simulink model "bike_model_v1_20190531_oldmodel_positionfeedback"  (R2016b)
settings: Solver=ode23s  StartTime=0.0  StopTime=sim_time  FixedStep=Ts_IMU  MaxStep=Ts  RelTol=1e-3
values from neighbouring files (symbols this model uses):
  A = [0      0            1 ... (first row only)    [bike_init_v1_20190528_oldmodel_positionfeedback_and_indicator.m]    (also in bike_init_v1_20190531_oldmodel_positionfeedback_and_indicator.m)
  A_kalman = [1 0 Ts 0; 0 1 0 Ts; 0 0 1 0; 0 0 0 1]    [bike_init_v1_20190528_oldmodel_positionfeedback_and_indicator.m]    (also in bike_init_v1_20190531_oldmodel_positionfeedback_and_indicator.m)
  a_real = b_real-0.77    (= 0.325)    [bike_init_v1_20190528_oldmodel_positionfeedback_and_indicator.m]    (also in bike_init_v1_20190531_oldmodel_positionfeedback_and_indicator.m)
  B = [0; 1; (a_real*v*sin(lambda_real))/(h_real*b_real)]    [bike_init_v1_20190528_oldmodel_positionfeedback_and_indicator.m]    (also in bike_init_v1_20190531_oldmodel_positionfeedback_and_indicator.m)
  B_kalman = [0 0 0 0; 0 0 0 0; 0 0 0 0; 0 0 0 0]    [bike_init_v1_20190528_oldmodel_positionfeedback_and_indicator.m]    (also in bike_init_v1_20190531_oldmodel_positionfeedback_and_indicator.m)
  b_model = 1.095    [bike_init_v1_20190528_oldmodel_positionfeedback_and_indicator.m]    (also in bike_init_v1_20190531_oldmodel_positionfeedback_and_indicator.m)
  b_real = 1.095    [bike_init_v1_20190528_oldmodel_positionfeedback_and_indicator.m]    (also in bike_init_v1_20190531_oldmodel_positionfeedback_and_indicator.m)
  C = eye(3)    [bike_init_v1_20190528_oldmodel_positionfeedback_and_indicator.m]    (also in bike_init_v1_20190531_oldmodel_positionfeedback_and_indicator.m)
  C_kalman = [1 0 0 0; 0 1 0 0; 0 0 1 0; 0 0 0 1]    [bike_init_v1_20190528_oldmodel_positionfeedback_and_indicator.m]    (also in bike_init_v1_20190531_oldmodel_positionfeedback_and_indicator.m)
  complementary = 0.985    [bike_init_v1_20190528_oldmodel_positionfeedback_and_indicator.m]    (also in bike_init_v1_20190531_oldmodel_positionfeedback_and_indicator.m)
  cumulative_dist_along_path = [0;cumsum(dist_from_vertex_to_vertex,1)]    [bike_init_v1_20190528_oldmodel_positionfeedback_and_indicator.m]    (also in bike_init_v1_20190531_oldmodel_positionfeedback_and_indicator.m)
  D = zeros(3,1)    [bike_init_v1_20190528_oldmodel_positionfeedback_and_indicator.m]    (also in bike_init_v1_20190531_oldmodel_positionfeedback_and_indicator.m)
  D_kalman = [0 0 0 0; 0 0 0 0; 0 0 0 0; 0 0 0 0]    [bike_init_v1_20190528_oldmodel_positionfeedback_and_indicator.m]    (also in bike_init_v1_20190531_oldmodel_positionfeedback_and_indicator.m)
  damp = 0.4    [bike_init_v1_20190528_oldmodel_positionfeedback_and_indicator.m]    (also in bike_init_v1_20190531_oldmodel_positionfeedback_and_indicator.m)
  Dead_Band = [0.055,-0.055,0.005]    [bike_init_v1_20190528_oldmodel_positionfeedback_and_indicator.m]    (also in bike_init_v1_20190531_oldmodel_positionfeedback_and_indicator.m)
  delay = 0.045    [bike_init_v1_20190528_oldmodel_positionfeedback_and_indicator.m]    (also in bike_init_v1_20190531_oldmodel_positionfeedback_and_indicator.m)
  delta_control = 1    [bike_init_v1_20190528_oldmodel_positionfeedback_and_indicator.m]    (also in bike_init_v1_20190531_oldmodel_positionfeedback_and_indicator.m)
  direct_control = 1    [bike_init_v1_20190528_oldmodel_positionfeedback_and_indicator.m]    (also in bike_init_v1_20190531_oldmodel_positionfeedback_and_indicator.m)
  filter_model = 1    [bike_init_v1_20190528_oldmodel_positionfeedback_and_indicator.m]    (also in bike_init_v1_20190531_oldmodel_positionfeedback_and_indicator.m)
  forward_motor_dynamics = 0    [bike_init_v1_20190528_oldmodel_positionfeedback_and_indicator.m]    (also in bike_init_v1_20190531_oldmodel_positionfeedback_and_indicator.m)
  fr_oscil = 1    [bike_init_v1_20190528_oldmodel_positionfeedback_and_indicator.m]    (also in bike_init_v1_20190531_oldmodel_positionfeedback_and_indicator.m)
  g = 9.81    [bike_init_v1_20190528_oldmodel_positionfeedback_and_indicator.m]    (also in bike_init_v1_20190531_oldmodel_positionfeedback_and_indicator.m)
  gain = 0.3    [bike_init_v1_20190528_oldmodel_positionfeedback_and_indicator.m]    (also in bike_init_v1_20190531_oldmodel_positionfeedback_and_indicator.m)
  h_real = 0.586    [bike_init_v1_20190528_oldmodel_positionfeedback_and_indicator.m]    (also in bike_init_v1_20190531_oldmodel_positionfeedback_and_indicator.m)
  IMU_height_model = 0.45    [bike_init_v1_20190528_oldmodel_positionfeedback_and_indicator.m]    (also in bike_init_v1_20190531_oldmodel_positionfeedback_and_indicator.m)
  IMU_height_real = 0.45    [bike_init_v1_20190528_oldmodel_positionfeedback_and_indicator.m]    (also in bike_init_v1_20190531_oldmodel_positionfeedback_and_indicator.m)
  initial_states = [deg2rad(0) deg2rad(0) deg2rad(0)]    [bike_init_v1_20190528_oldmodel_positionfeedback_and_indicator.m]    (also in bike_init_v1_20190531_oldmodel_positionfeedback_and_indicator.m = [deg2rad(2) deg2rad(0) deg2rad(0)])
  initial_x = path_x(1)+x_ini_diff    [bike_init_v1_20190528_oldmodel_positionfeedback_and_indicator.m]    (also in bike_init_v1_20190531_oldmodel_positionfeedback_and_indicator.m = 0)
  initial_y = radius+y_ini_diff    (= 20)    [bike_init_v1_20190528_oldmodel_positionfeedback_and_indicator.m]    (also in bike_init_v1_20190531_oldmodel_positionfeedback_and_indicator.m = 0)
  input_velocity = 7    [bike_init_v1_20190528_oldmodel_positionfeedback_and_indicator.m]    (also in bike_init_v1_20190531_oldmodel_positionfeedback_and_indicator.m = 3)
  K_full_dis = zeros(length(velocity_lqr),3)    [bike_init_v1_20190528_oldmodel_positionfeedback_and_indicator.m]    (also in bike_init_v1_20190531_oldmodel_positionfeedback_and_indicator.m)
  lambda_model = deg2rad(70)    [bike_init_v1_20190528_oldmodel_positionfeedback_and_indicator.m]    (also in bike_init_v1_20190531_oldmodel_positionfeedback_and_indicator.m)
  lambda_real = deg2rad(70)    [bike_init_v1_20190528_oldmodel_positionfeedback_and_indicator.m]    (also in bike_init_v1_20190531_oldmodel_positionfeedback_and_indicator.m)
  lat_control = 1    [bike_init_v1_20190528_oldmodel_positionfeedback_and_indicator.m]    (also in bike_init_v1_20190531_oldmodel_positionfeedback_and_indicator.m)
  look_ahead = 0    [bike_init_v1_20190528_oldmodel_positionfeedback_and_indicator.m]    (also in bike_init_v1_20190531_oldmodel_positionfeedback_and_indicator.m)
  max_handlebar = 40*(pi/180)    (= 0.698131700798)    [bike_init_v1_20190528_oldmodel_positionfeedback_and_indicator.m]    (also in bike_init_v1_20190531_oldmodel_positionfeedback_and_indicator.m)
  max_roll = pi/2    (= 1.57079632679)    [bike_init_v1_20190528_oldmodel_positionfeedback_and_indicator.m]    (also in bike_init_v1_20190531_oldmodel_positionfeedback_and_indicator.m)
  max_steering_motor_acc = inf    [bike_init_v1_20190528_oldmodel_positionfeedback_and_indicator.m]    (also in bike_init_v1_20190531_oldmodel_positionfeedback_and_indicator.m)
  max_steering_motor_speed = 7.5    [bike_init_v1_20190528_oldmodel_positionfeedback_and_indicator.m]    (also in bike_init_v1_20190531_oldmodel_positionfeedback_and_indicator.m)
  min_handlebar = -max_handlebar    (= -0.698131700798)    [bike_init_v1_20190528_oldmodel_positionfeedback_and_indicator.m]    (also in bike_init_v1_20190531_oldmodel_positionfeedback_and_indicator.m)
  min_roll = - max_roll    (= -1.57079632679)    [bike_init_v1_20190528_oldmodel_positionfeedback_and_indicator.m]    (also in bike_init_v1_20190531_oldmodel_positionfeedback_and_indicator.m)
  min_steering_motor_acc = -inf    [bike_init_v1_20190528_oldmodel_positionfeedback_and_indicator.m]    (also in bike_init_v1_20190531_oldmodel_positionfeedback_and_indicator.m)
  min_steering_motor_speed = -7.5    [bike_init_v1_20190528_oldmodel_positionfeedback_and_indicator.m]    (also in bike_init_v1_20190531_oldmodel_positionfeedback_and_indicator.m)
  noise = 1    [bike_init_v1_20190528_oldmodel_positionfeedback_and_indicator.m]    (also in bike_init_v1_20190531_oldmodel_positionfeedback_and_indicator.m)
  noise_encoder = 1e-7    (= 1e-07)    [bike_init_v1_20190528_oldmodel_positionfeedback_and_indicator.m]    (also in bike_init_v1_20190531_oldmodel_positionfeedback_and_indicator.m)
  noise_hall = 0.01    [bike_init_v1_20190528_oldmodel_positionfeedback_and_indicator.m]    (also in bike_init_v1_20190531_oldmodel_positionfeedback_and_indicator.m = 0.0031)
  noise_pos_meas = 0.51    [bike_init_v1_20190528_oldmodel_positionfeedback_and_indicator.m]    (also in bike_init_v1_20190531_oldmodel_positionfeedback_and_indicator.m)
  oscillations_roll = 0    [bike_init_v1_20190528_oldmodel_positionfeedback_and_indicator.m]    (also in bike_init_v1_20190531_oldmodel_positionfeedback_and_indicator.m)
  oscillations_steer = 0    [bike_init_v1_20190528_oldmodel_positionfeedback_and_indicator.m]    (also in bike_init_v1_20190531_oldmodel_positionfeedback_and_indicator.m)
  parameters_model = [g h_model b_model a_model lambda_model c_model]    [bike_init_v1_20190528_oldmodel_positionfeedback_and_indicator.m]    (also in bike_init_v1_20190531_oldmodel_positionfeedback_and_indicator.m)
  parameters_real = [g h_real b_real a_real lambda_real c_real]    [bike_init_v1_20190528_oldmodel_positionfeedback_and_indicator.m]    (also in bike_init_v1_20190531_oldmodel_positionfeedback_and_indicator.m)
  path_tracking = 0    [bike_init_v1_20190528_oldmodel_positionfeedback_and_indicator.m]    (also in bike_init_v1_20190531_oldmodel_positionfeedback_and_indicator.m)
  path_x = [path_x1 path_x2 path_x3]    [bike_init_v1_20190528_oldmodel_positionfeedback_and_indicator.m]    (also in bike_init_v1_20190531_oldmodel_positionfeedback_and_indicator.m)
  path_y = [path_y1 path_y2 path_y3]    [bike_init_v1_20190528_oldmodel_positionfeedback_and_indicator.m]    (also in bike_init_v1_20190531_oldmodel_positionfeedback_and_indicator.m)
  plant_model = 1    [bike_init_v1_20190528_oldmodel_positionfeedback_and_indicator.m]    (also in bike_init_v1_20190531_oldmodel_positionfeedback_and_indicator.m)
  R_kalman = [noise_pos_meas 0 0 0; 0 noise_pos_meas 0 0; 0 0 noise_hall 0; 0 0 0 noise_hall]    [bike_init_v1_20190528_oldmodel_positionfeedback_and_indicator.m]    (also in bike_init_v1_20190531_oldmodel_positionfeedback_and_indicator.m)
  roll_rate_coef = 0.9    [bike_init_v1_20190528_oldmodel_positionfeedback_and_indicator.m]    (also in bike_init_v1_20190531_oldmodel_positionfeedback_and_indicator.m)
  steering_motor_limitations = 1    [bike_init_v1_20190528_oldmodel_positionfeedback_and_indicator.m]    (also in bike_init_v1_20190531_oldmodel_positionfeedback_and_indicator.m)
  sys_con = ss(A,B,C,D)    [bike_init_v1_20190528_oldmodel_positionfeedback_and_indicator.m]    (also in bike_init_v1_20190531_oldmodel_positionfeedback_and_indicator.m)
  sys_dis = c2d(sys_con,Ts)    [bike_init_v1_20190528_oldmodel_positionfeedback_and_indicator.m]    (also in bike_init_v1_20190531_oldmodel_positionfeedback_and_indicator.m)
  Ts = 0.04    [bike_init_v1_20190528_oldmodel_positionfeedback_and_indicator.m]    (also in bike_init_v1_20190531_oldmodel_positionfeedback_and_indicator.m)
  Ts_IMU = 0.04    [bike_init_v1_20190528_oldmodel_positionfeedback_and_indicator.m]    (also in bike_init_v1_20190531_oldmodel_positionfeedback_and_indicator.m)
  velocity_lqr = [velocity_lqr-0.1 velocity_lqr velocity_lqr+0.1]    [bike_init_v1_20190528_oldmodel_positionfeedback_and_indicator.m]    (also in bike_init_v1_20190531_oldmodel_positionfeedback_and_indicator.m)
  velocity_wave_amp = 0.5    [bike_init_v1_20190528_oldmodel_positionfeedback_and_indicator.m]    (also in bike_init_v1_20190531_oldmodel_positionfeedback_and_indicator.m)
  velocity_wave_freq = 0.3*2*pi    (= 1.88495559215)    [bike_init_v1_20190528_oldmodel_positionfeedback_and_indicator.m]    (also in bike_init_v1_20190531_oldmodel_positionfeedback_and_indicator.m)
undefined symbols (not defined in the file or in its folder): Continuous, curvature, Time
libraries: simulink x13, mpclib x2, dspsigops x2, simulink_extras x1, ctrlSharedLib x1
(part 2 of 2)

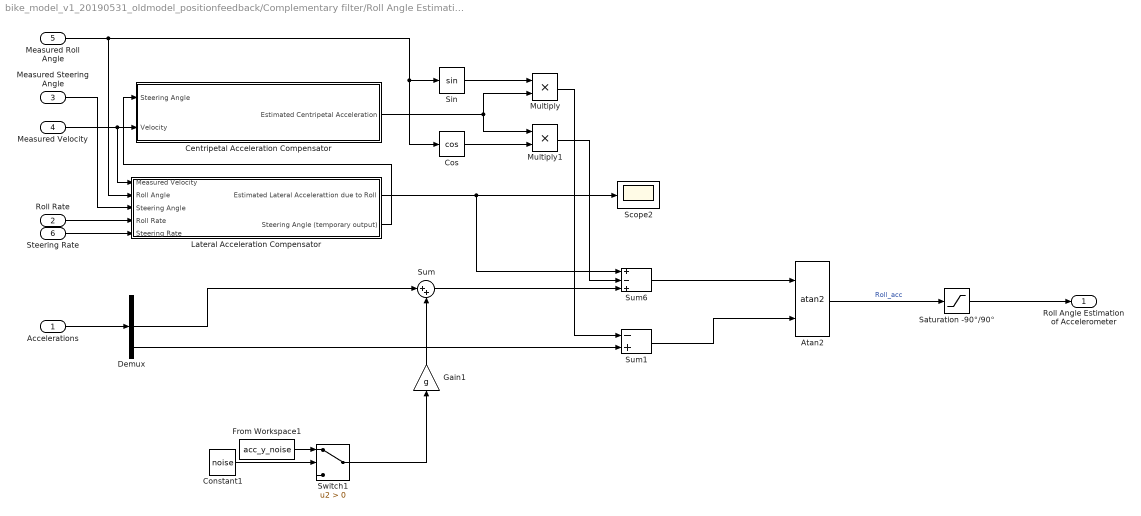
== system bike_model_v1_20190531_oldmodel_positionfeedback/Complementary filter/Roll Angle Estimation of Accelerometer ==
  Accelerations : Inport
  Roll Rate : Inport  Port=2
  Measured Steering Angle : Inport  Port=3
  Measured Velocity : Inport  Port=4
  Measured Roll Angle : Inport  Port=5
  Steering Rate : Inport  Port=6
  Atan2 : Trigonometry  Operator=atan2
  Centripetal Acceleration Compensator : Subsystem
  Constant1 : Constant  Value=noise
  Cos : Trigonometry  Operator=cos
  Demux : Demux  Outputs=3
  From Workspace1 : FromWorkspace  VariableName=acc_y_noise  SampleTime=0
  Gain1 : Gain  Gain=g
  Lateral Acceleration Compensator : Subsystem
  Multiply : Product
  Multiply1 : Product
  Saturation -90°/90° : Saturate  UpperLimit=max_roll  LowerLimit=min_roll
  Scope2 : Scope
  Sin : Trigonometry
  Sum : Sum  Inputs=|++
  Sum1 : Sum  Inputs=-+
  Sum6 : Sum  Inputs=+-+
  Switch1 : Switch  Criteria=u2 > Threshold
  Roll Angle Estimation of Accelerometer : Outport
  wires:
  Sum1/1 -> Atan2/2
  Lateral Acceleration Compensator/1(Estimated Lateral Accelerattion due to Roll) -> Scope2/1, Sum6/1
  Atan2/1 -> Saturation -90°/90°/1  "Roll_acc"
  Roll Rate/1 -> Lateral Acceleration Compensator/4(Roll Rate)
  Demux/2 -> Sum/1
  Accelerations/1 -> Demux/1
  Measured Velocity/1 -> Lateral Acceleration Compensator/1(Measured Velocity), Centripetal Acceleration Compensator/2(Velocity)
  Measured Steering Angle/1 -> Lateral Acceleration Compensator/3(Steering Angle)
  Centripetal Acceleration Compensator/1(Estimated Centripetal Acceleration) -> Multiply/2, Multiply1/1
  Measured Roll Angle/1 -> Lateral Acceleration Compensator/2(Roll Angle), Sin/1, Cos/1
  Cos/1 -> Multiply1/2
  Sin/1 -> Multiply/1
  Multiply1/1 -> Sum6/2
  Demux/3 -> Sum1/2
  Multiply/1 -> Sum1/1
  Steering Rate/1 -> Lateral Acceleration Compensator/5(Steering Rate)
  Sum6/1 -> Atan2/1
  Lateral Acceleration Compensator/2(Steering Angle (temporary output)) -> Centripetal Acceleration Compensator/1(Steering Angle)
  From Workspace1/1 -> Switch1/1
  Constant1/1 -> Switch1/2
  Sum/1 -> Sum6/3
  Switch1/1 -> Gain1/1
  Gain1/1 -> Sum/2
  Saturation -90°/90°/1 -> Roll Angle Estimation of Accelerometer/1

== system bike_model_v1_20190531_oldmodel_positionfeedback/Global Angles and Coordinates Calculator - Position/Measured Bike Angles to Global Angles ==
  Velocity : Inport
  Steering Angle : Inport  Port=2
  " Bike Parameters Model " : Constant  Value=parameters_model
  Integrator : Integrator
  MATLAB Function : MATLAB Function  TreatAsAtomicUnit=on
  To Workspace6 : ToWorkspace  VariableName=PSI  SaveFormat=Timeseries  SampleTime=Ts
  To Workspace7 : ToWorkspace  VariableName=BETA  SaveFormat=Timeseries  SampleTime=Ts
  psi : Outport
  beta : Outport  Port=2
  wires:
  MATLAB Function/2(beta) -> beta/1, To Workspace7/1
  MATLAB Function/1(psi_d) -> Integrator/1
  Integrator/1 -> To Workspace6/1, psi/1
  " Bike Parameters Model "/1 -> MATLAB Function/2(parameters_model)
  Steering Angle/1 -> MATLAB Function/3(delta)
  Velocity/1 -> MATLAB Function/1(v)

== system bike_model_v1_20190531_oldmodel_positionfeedback/Global Angles and Coordinates Calculator - Position/Measured Global Angles to Global Coordinates ==
  Velocity : Inport
  Psi : Inport  Port=2
  Beta : Inport  Port=3
  Constant : Constant  Value=initial_y
  Constant1 : Constant  Value=initial_x
  Integrator1 : Integrator
  Integrator2 : Integrator
  MATLAB Function1 : MATLAB Function  TreatAsAtomicUnit=on
  Mux : Mux  Inputs=2
  Sum : Sum  Inputs=|++
  Sum1 : Sum  Inputs=++|
  "Position (X, Y)" : Outport
  wires:
  MATLAB Function1/2(Ydot) -> Integrator2/1  "Ydot"
  MATLAB Function1/1(Xdot) -> Integrator1/1  "Xdot"
  Psi/1 -> MATLAB Function1/2(psi)
  Beta/1 -> MATLAB Function1/3(beta)
  Velocity/1 -> MATLAB Function1/1(v)
  Integrator2/1 -> Sum/1
  Constant/1 -> Sum/2
  Sum/1 -> Mux/2
  Integrator1/1 -> Sum1/2
  Sum1/1 -> Mux/1
  Constant1/1 -> Sum1/1
  Mux/1 -> "Position (X, Y)"/1

== system bike_model_v1_20190531_oldmodel_positionfeedback/Global Angles and Coordinates Calculator - Velocity/Measured Bike Angles to Global Angles ==
  note: Verification of the equivalence of the calculus for Beta estimation
  Velocity : Inport
  Steering Angle : Inport  Port=2
  Gain : Gain  Gain=1/b_model
  Integrator : Integrator
  MATLAB Function : MATLAB Function  TreatAsAtomicUnit=on
  Multiply : Product
  Parameters : Constant  Value=parameters_model
  Scope : Scope  NumInputPorts=2
  Tan : Trigonometry  Operator=tan
  psi : Outport
  beta : Outport  Port=2
  wires:
  Integrator/1 -> psi/1
  MATLAB Function/1(psi_d) -> Scope/1, Integrator/1
  Steering Angle/1 -> Tan/1, MATLAB Function/3(delta)
  Parameters/1 -> MATLAB Function/2(parameters_model)
  Velocity/1 -> Multiply/1, MATLAB Function/1(v)
  MATLAB Function/2(beta) -> beta/1
  Tan/1 -> Multiply/2
  Multiply/1 -> Gain/1
  Gain/1 -> Scope/2

== system bike_model_v1_20190531_oldmodel_positionfeedback/Global Angles and Coordinates Calculator - Velocity/Measured Global Angles to Global Coordinates ==
  Velocity : Inport
  Psi : Inport  Port=2
  Beta : Inport  Port=3
  MATLAB Function1 : MATLAB Function  TreatAsAtomicUnit=on
  Mux1 : Mux  Inputs=2
  "Velocity (Xdot, Ydot)" : Outport
  wires:
  MATLAB Function1/2(Ydot) -> Mux1/2  "Ydot"
  MATLAB Function1/1(Xdot) -> Mux1/1  "Xdot"
  Psi/1 -> MATLAB Function1/2(psi)
  Beta/1 -> MATLAB Function1/3(beta)
  Velocity/1 -> MATLAB Function1/1(v)
  Mux1/1 -> "Velocity (Xdot, Ydot)"/1

== system bike_model_v1_20190531_oldmodel_positionfeedback/IMU/IMU ==
  Lateral Acceleration : Inport
  Centripetal Acceleration : Inport  Port=2
  True Velocity : Inport  Port=3
  True Roll Angle : Inport  Port=4
  Measured Steering Angle : Inport  Port=5
  IMU Accelerometer : Subsystem
  IMU Gyroscope : Subsystem
  Accelerations : Outport
  Roll Rates : Outport  Port=2
  wires:
  Lateral Acceleration/1 -> IMU Accelerometer/1(Lateral Acceleration of the IMU due to Roll)
  Centripetal Acceleration/1 -> IMU Accelerometer/2(Centripetal Acceleration due to Path Curvature)
  True Roll Angle/1 -> IMU Gyroscope/2(True Roll Angle), IMU Accelerometer/4(True Roll Angle)
  IMU Accelerometer/1(Accelerations) -> Accelerations/1
  IMU Gyroscope/1(Roll rates) -> Roll Rates/1
  True Velocity/1 -> IMU Gyroscope/1(True Velocity), IMU Accelerometer/3(True Velocity)
  Measured Steering Angle/1 -> IMU Gyroscope/3(Measured Steering Angle)

== system bike_model_v1_20190531_oldmodel_positionfeedback/Path Tracking Controllers/Lateral Error ==
  Psi Sigma : Inport
  Position Error (X,Y) : Inport  Port=2
  Cos : Trigonometry  Operator=cos
  Demux : Demux  Outputs=2
  Product : Product
  Product1 : Product
  Sin : Trigonometry
  Sum : Sum  Inputs=+-|
  To Workspace4 : ToWorkspace  VariableName=LAT_ERR  SaveFormat=Timeseries  SampleTime=Ts
  Lateral Error : Outport
  wires:
  Cos/1 -> Product/2
  Sin/1 -> Product1/1
  Psi Sigma/1 -> Cos/1, Sin/1
  Product1/1 -> Sum/2
  Product/1 -> Sum/1
  Sum/1 -> To Workspace4/1, Lateral Error/1  "Lateral Error"
  Demux/1 -> Product1/2  "X Position Error"
  Demux/2 -> Product/1  "Y Position Error"
  Position Error (X,Y)/1 -> Demux/1

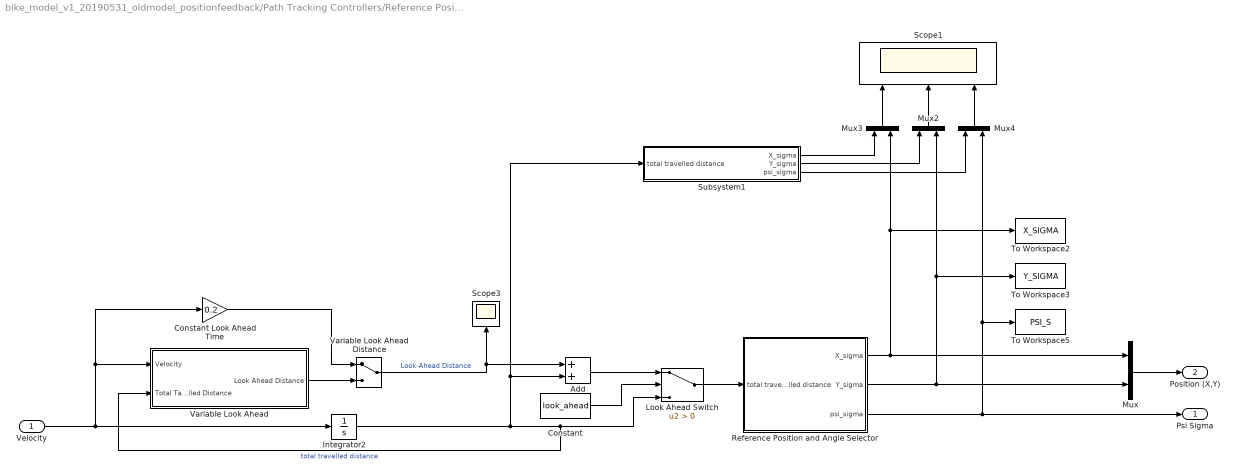
== system bike_model_v1_20190531_oldmodel_positionfeedback/Path Tracking Controllers/Reference Position and Direction in Global CS with variable Look Ahead ==
  Velocity : Inport
  Add : Sum
  Constant : Constant  Value=look_ahead
  Constant Look Ahead Time : Gain  Gain=0.2
  Integrator2 : Integrator
  Look Ahead Switch : Switch  Criteria=u2 > Threshold
  Mux{,2..4} (4 alike) : Mux  Inputs=2
  Reference Position and Angle Selector : Subsystem
  Scope1 : Scope  NumInputPorts=3
  Scope3 : Scope
  Subsystem1 : Subsystem
  To Workspace2 : ToWorkspace  VariableName=X_SIGMA  SaveFormat=Timeseries  SampleTime=Ts
  To Workspace3 : ToWorkspace  VariableName=Y_SIGMA  SaveFormat=Timeseries  SampleTime=Ts
  To Workspace5 : ToWorkspace  VariableName=PSI_S  SaveFormat=Timeseries  SampleTime=Ts
  Variable Look Ahead Distance : ManualSwitch
  Variable Look Ahead : Subsystem
  Psi Sigma : Outport
  Position (X,Y) : Outport  Port=2
  wires:
  Constant Look Ahead Time/1 -> Variable Look Ahead Distance/1
  Reference Position and Angle Selector/3(psi_sigma) -> To Workspace5/1, Mux4/2, Psi Sigma/1
  Mux3/1 -> Scope1/1
  Subsystem1/3(psi_sigma) -> Mux4/1
  Mux2/1 -> Scope1/2
  Mux4/1 -> Scope1/3
  Velocity/1 -> Integrator2/1, Constant Look Ahead Time/1, Variable Look Ahead/1(Velocity)
  Add/1 -> Look Ahead Switch/1
  Reference Position and Angle Selector/2(Y_sigma) -> To Workspace3/1, Mux2/2, Mux/2
  Look Ahead Switch/1 -> Reference Position and Angle Selector/1(total travelled distance)
  Subsystem1/2(Y_sigma) -> Mux2/1
  Integrator2/1 -> Variable Look Ahead/2(Total Tavelled Distance), Look Ahead Switch/3, Subsystem1/1(total travelled distance), Add/2  "total travelled distance"
  Subsystem1/1(X_sigma) -> Mux3/1
  Reference Position and Angle Selector/1(X_sigma) -> Mux3/2, To Workspace2/1, Mux/1
  Variable Look Ahead Distance/1 -> Scope3/1, Add/1  "Look-Ahead Distance"
  Constant/1 -> Look Ahead Switch/2
  Mux/1 -> Position (X,Y)/1
  Variable Look Ahead/1(Look Ahead Distance) -> Variable Look Ahead Distance/2

== system bike_model_v1_20190531_oldmodel_positionfeedback/Physical Bike/Centripetal Acceleration Calculator ==
  True Steering Angle : Inport
  True Velocity : Inport  Port=2
  Divide : Product  Inputs=*/
  Gain : Gain  Gain=sin(lambda_real)
  Multiply : Product
  Square : Math  Operator=square  SaturateOnIntegerOverflow=on
  Tan : Trigonometry  Operator=tan
  b Real Bike : Constant  Value=b_real
  Centripetal Acceleration : Outport
  wires:
  True Velocity/1 -> Square/1
  Square/1 -> Divide/1
  b Real Bike/1 -> Divide/2
  True Steering Angle/1 -> Gain/1
  Divide/1 -> Multiply/1
  Tan/1 -> Multiply/2
  Multiply/1 -> Centripetal Acceleration/1
  Gain/1 -> Tan/1

== system bike_model_v1_20190531_oldmodel_positionfeedback/Physical Bike/Check Phi Limits ==
  x : Inport
  Roll Lower Bound : simulink/Model Verification/Check Static  Lower Bound  Description=min_roll <= u  min=min_roll  min_included=on  enabled=on  stopWhenAssertionFail=on  export=off  icon=graphic
  Roll Upper Bound : simulink/Model Verification/Check Static  Upper Bound  Description=u <= max_roll  max=max_roll  max_included=on  enabled=on  stopWhenAssertionFail=on  export=off  icon=graphic
  wires:
  x/1 -> Roll Lower Bound/1, Roll Upper Bound/1  "Roll Angle"

== system bike_model_v1_20190531_oldmodel_positionfeedback/Physical Bike/Lateral Acceleration (due to Roll) Calculator ==
  Roll Acceleration : Inport
  Constant3 : Constant  Value=IMU_height_real
  Multiply : Product
  Lateral Acceleration : Outport
  wires:
  Multiply/1 -> Lateral Acceleration/1
  Constant3/1 -> Multiply/1
  Roll Acceleration/1 -> Multiply/2

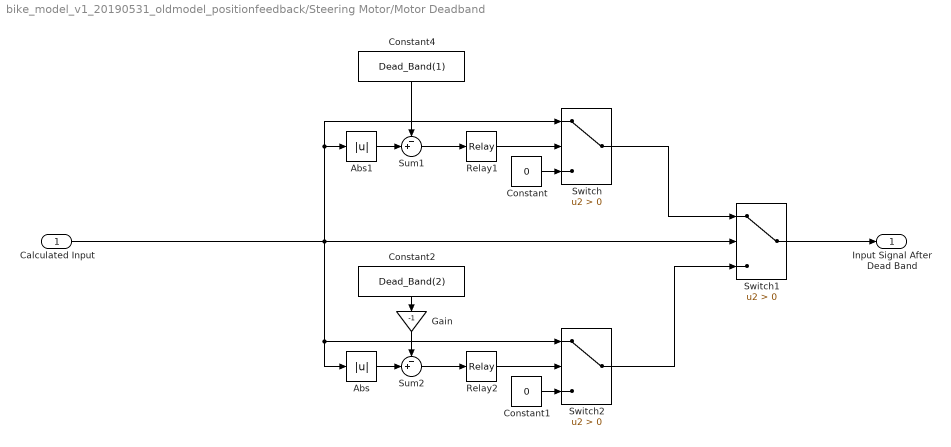
== system bike_model_v1_20190531_oldmodel_positionfeedback/Steering Motor/Motor Deadband ==
  Calculated Input : Inport
  Abs : Abs
  Abs1 : Abs
  Constant : Constant  Value=0  SampleTime=Ts
  Constant1 : Constant  Value=0  SampleTime=Ts
  Constant2 : Constant  Value=Dead_Band(2)  SampleTime=Ts
  Constant4 : Constant  Value=Dead_Band(1)  SampleTime=Ts
  Gain : Gain  Gain=-1
  Relay1 : Relay  OnSwitchValue=Dead_Band(3)  OffSwitchValue=-Dead_Band(3)
  Relay2 : Relay  OnSwitchValue=Dead_Band(3)  OffSwitchValue=-Dead_Band(3)
  Sum1 : Sum  Inputs=-+|
  Sum2 : Sum  Inputs=-+|
  Switch : Switch  Criteria=u2 > Threshold
  Switch1 : Switch  Criteria=u2 > Threshold
  Switch2 : Switch  Criteria=u2 > Threshold
  Input Signal After Dead Band : Outport
  wires:
  Constant4/1 -> Sum1/1
  Sum1/1 -> Relay1/1
  Relay1/1 -> Switch/2
  Switch/1 -> Switch1/1
  Constant/1 -> Switch/3
  Switch1/1 -> Input Signal After Dead Band/1
  Switch2/1 -> Switch1/3
  Constant1/1 -> Switch2/3
  Gain/1 -> Sum2/1
  Calculated Input/1 -> Abs/1, Switch2/1, Abs1/1, Switch/1, Switch1/2
  Sum2/1 -> Relay2/1
  Relay2/1 -> Switch2/2
  Abs/1 -> Sum2/2
  Abs1/1 -> Sum1/2
  Constant2/1 -> Gain/1

== system bike_model_v1_20190531_oldmodel_positionfeedback/Steering Motor/Velocity Saturation wrt Max and Min Handle Bar Angles ==
  Reference Velocity : Inport
  States : Inport  Port=2
  AND : Logic  IconShape=distinctive  AllPortsSameDT=off  OutDataTypeStr=boolean
  AND1 : Logic  IconShape=distinctive  AllPortsSameDT=off  OutDataTypeStr=boolean
  Compare To Constant : simulink/Logic and Bit Operations/Compare To Constant  relop=>=  const=max_handlebar  OutDataTypeStr=boolean
  Compare To Constant1 : simulink/Logic and Bit Operations/Compare To Constant  relop=<=  const=min_handlebar  OutDataTypeStr=boolean
  Compare To Zero : simulink/Logic and Bit Operations/Compare To Zero  relop=>=  OutDataTypeStr=boolean
  Compare To Zero1 : simulink/Logic and Bit Operations/Compare To Zero  relop=<=  OutDataTypeStr=boolean
  Constant : Constant  Value=0
  Demux : Demux  Outputs=3
  OR : Logic  Operator=OR  IconShape=distinctive  AllPortsSameDT=off  OutDataTypeStr=boolean
  Switch : Switch  Criteria=u2 > Threshold
  Output Steering Velocity : Outport
  wires:
  Switch/1 -> Output Steering Velocity/1
  Constant/1 -> Switch/1
  States/1 -> Demux/1
  Compare To Constant/1 -> AND/2
  OR/1 -> Switch/2
  Reference Velocity/1 -> Switch/3, Compare To Zero1/1, Compare To Zero/1
  Compare To Constant1/1 -> AND1/1
  AND1/1 -> OR/2
  Demux/2 -> Compare To Constant/1, Compare To Constant1/1
  AND/1 -> OR/1
  Compare To Zero1/1 -> AND1/2
  Compare To Zero/1 -> AND/1

== system bike_model_v1_20190531_oldmodel_positionfeedback/Complementary filter/Roll Angle Estimation of Accelerometer/Centripetal Acceleration Compensator ==
  Steering Angle : Inport
  Velocity : Inport  Port=2
  Bike Model b : Constant  Value=b_model
  Divide : Product  Inputs=*/
  Gain : Gain  Gain=sin(lambda_model)
  Multiply : Product
  Square : Math  Operator=square  SaturateOnIntegerOverflow=on
  Tan : Trigonometry  Operator=tan
  Estimated Centripetal Acceleration : Outport
  wires:
  Velocity/1 -> Square/1
  Square/1 -> Divide/1
  Bike Model b/1 -> Divide/2
  Steering Angle/1 -> Gain/1
  Divide/1 -> Multiply/1
  Tan/1 -> Multiply/2
  Multiply/1 -> Estimated Centripetal Acceleration/1
  Gain/1 -> Tan/1

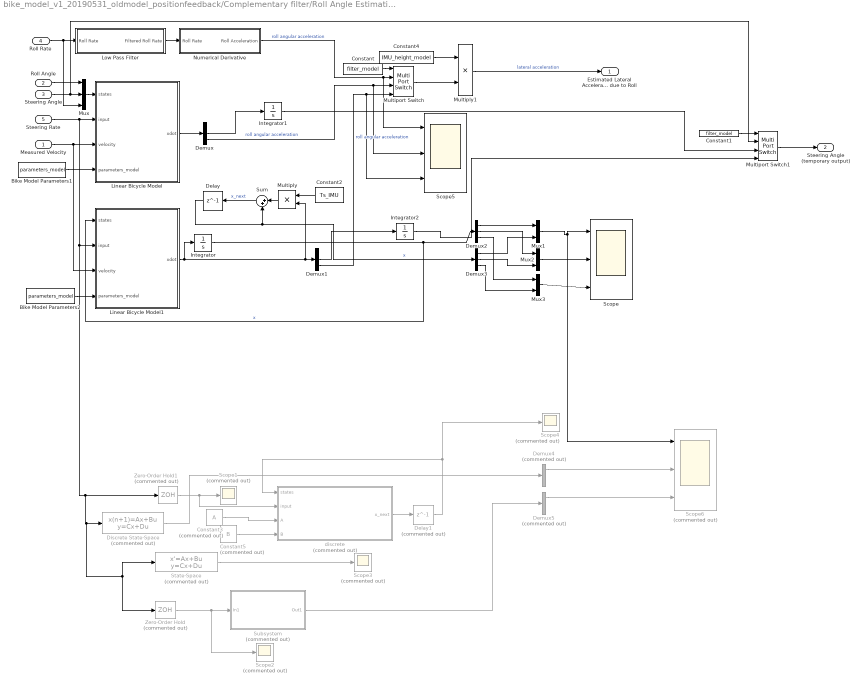
== system bike_model_v1_20190531_oldmodel_positionfeedback/Complementary filter/Roll Angle Estimation of Accelerometer/Lateral Acceleration Compensator ==
  Measured Velocity : Inport
  Roll Angle : Inport  Port=2
  Steering Angle : Inport  Port=3
  Roll Rate : Inport  Port=4
  Steering Rate : Inport  Port=5
  Bike Model Parameters1 : Constant  Value=parameters_model
  Bike Model Parameters2 : Constant  Value=parameters_model
  Constant : Constant  Value=filter_model
  Constant1 : Constant  Value=filter_model
  Constant2 : Constant  Value=Ts_IMU  SampleTime=Ts_IMU
  Constant3 : Constant  Commented=on  Value=A
  Constant4 : Constant  Value=IMU_height_model
  Constant5 : Constant  Commented=on  Value=B
  Delay : Delay  DelayLength=1  InitialCondition=[0 0 0]  SampleTime=Ts_IMU
  Delay1 : Delay  Commented=on  DelayLength=1  InitialCondition=[0 0 0]  SampleTime=Ts_IMU
  Demux{,1..3} (4 alike) : Demux  Outputs=3
  Demux4 : Demux  Commented=on  Outputs=3
  Demux5 : Demux  Commented=on  Outputs=3
  Discrete State-Space : DiscreteStateSpace  Commented=on  A=A  B=B  C=eye(3,3)  D=zeros(3,1)  X0=[0 0 0]  SampleTime=Ts_IMU
  Integrator : Integrator  InitialCondition=initial_states
  Integrator1 : Integrator  InitialCondition=initial_states(2)
  Integrator2 : Integrator  InitialCondition=initial_states(2)
  Linear Bicycle Model : MATLAB Function  TreatAsAtomicUnit=on
  Linear Bicycle Model1 : MATLAB Function  TreatAsAtomicUnit=on
  Low Pass Filter : Subsystem
  Multiply : Product
  Multiply1 : Product
  Multiport Switch : MultiPortSwitch
  Multiport Switch1 : MultiPortSwitch
  Mux : Mux  Inputs=3
  Mux1 : Mux  Inputs=2
  Mux2 : Mux  Inputs=2
  Mux3 : Mux  Inputs=2
  Numerical Derivative : Subsystem
  Scope : Scope  NumInputPorts=3
  Scope{1..4} (4 alike) : Scope  Commented=on
  Scope5 : Scope  NumInputPorts=3
  Scope6 : Scope  Commented=on  NumInputPorts=3
  State-Space : StateSpace  Commented=on  A=sys_con.A  B=sys_con.B  C=eye(3,3)  D=zeros(3,1)  X0=[0 0 0]
  Subsystem : Subsystem  Commented=on  TreatAsAtomicUnit=on  SystemSampleTime=Ts_IMU
  Sum : Sum  Inputs=|++
  Zero-Order Hold : ZeroOrderHold  Commented=on  SampleTime=Ts_IMU
  Zero-Order Hold1 : ZeroOrderHold  Commented=on  SampleTime=Ts_IMU
  discrete : MATLAB Function  Commented=on  TreatAsAtomicUnit=on
  Estimated Lateral Accelerattion due to Roll : Outport
  Steering Angle (temporary output) : Outport  Port=2
  wires:
  Numerical Derivative/1(Roll Acceleration) -> Scope5/1, Multiport Switch/2  "roll angular acceleration"
  Roll Rate/1 -> Mux/3, Low Pass Filter/1(Roll Rate)
  Constant4/1 -> Multiply1/1
  Multiply1/1 -> Estimated Lateral Accelerattion due to Roll/1  "lateral acceleration"
  Low Pass Filter/1(Filtered Roll Rate) -> Numerical Derivative/1(Roll Rate)
  Linear Bicycle Model/1(xdot) -> Demux/1
  Demux/3 -> Scope5/2, Multiport Switch/3  "roll angular acceleration"
  Bike Model Parameters1/1 -> Linear Bicycle Model/4(parameters_model)
  Measured Velocity/1 -> Linear Bicycle Model1/3(velocity), Linear Bicycle Model/3(velocity)
  Mux/1 -> Linear Bicycle Model/1(states)
  Roll Angle/1 -> Mux/1
  Steering Angle/1 -> Multiport Switch1/2, Mux/2
  Constant/1 -> Multiport Switch/1
  Multiport Switch/1 -> Multiply1/2
  Demux1/3 -> Scope5/3, Multiport Switch/4  "roll angular acceleration"
  Bike Model Parameters2/1 -> Linear Bicycle Model1/4(parameters_model)
  Delay/1 -> Demux3/1, Sum/2  "x"
  Multiply/1 -> Sum/1
  Constant2/1 -> Multiply/1
  Integrator/1 -> Linear Bicycle Model1/1(states), Demux2/1  "x"
  Demux2/1 -> Mux1/1
  Demux3/1 -> Mux1/2
  Demux2/2 -> Mux2/1
  Demux3/2 -> Mux2/2
  Demux2/3 -> Mux3/1
  Demux3/3 -> Mux3/2
  Mux2/1 -> Scope/2
  Mux1/1 -> Scope6/1, Scope/1
  Mux3/1 -> Scope/3
  Linear Bicycle Model1/1(xdot) -> Multiply/2, Demux1/1, Integrator/1
  State-Space/1 -> Scope3/1
  Delay1/1 -> Scope4/1, discrete/1(states)
  Zero-Order Hold/1 -> Scope2/1, Subsystem/1(In1)
  discrete/1(x_next) -> Delay1/1
  Constant5/1 -> discrete/4(B)
  Constant3/1 -> discrete/3(A)
  Sum/1 -> Delay/1  "x_next"
  Zero-Order Hold1/1 -> discrete/2(input), Scope1/1
  Multiport Switch1/1 -> Steering Angle (temporary output)/1
  Constant1/1 -> Multiport Switch1/1
  Steering Rate/1 -> Zero-Order Hold/1, State-Space/1, Discrete State-Space/1, Zero-Order Hold1/1, Linear Bicycle Model1/2(input), Linear Bicycle Model/2(input)
  Integrator1/1 -> Multiport Switch1/3
  Demux/2 -> Integrator1/1
  Demux1/2 -> Integrator2/1
  Integrator2/1 -> Multiport Switch1/4
  Demux4/1 -> Scope6/2
  Demux5/1 -> Scope6/3
  Discrete State-Space/1 -> Demux4/1
  Subsystem/1(Out1) -> Demux5/1

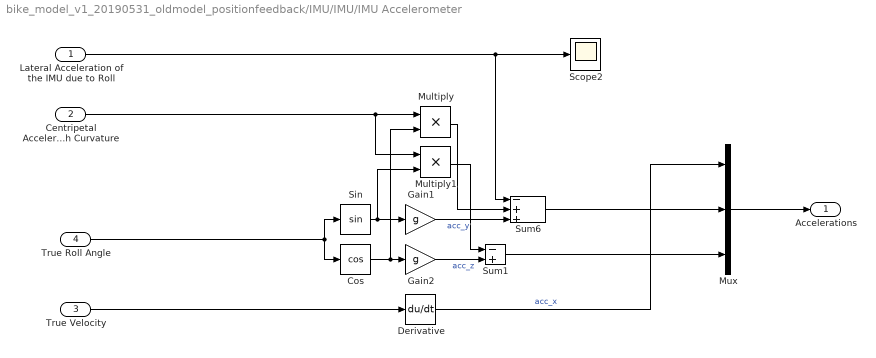
== system bike_model_v1_20190531_oldmodel_positionfeedback/IMU/IMU/IMU Accelerometer ==
  Lateral Acceleration of the IMU due to Roll : Inport
  Centripetal Acceleration due to Path Curvature : Inport  Port=2
  True Velocity : Inport  Port=3
  True Roll Angle : Inport  Port=4
  Cos : Trigonometry  Operator=cos
  Derivative : Derivative  CoefficientInTFapproximation=-1
  Gain1 : Gain  Gain=g
  Gain2 : Gain  Gain=g
  Multiply : Product
  Multiply1 : Product
  Mux : Mux  Inputs=3
  Scope2 : Scope
  Sin : Trigonometry
  Sum1 : Sum  Inputs=-+
  Sum6 : Sum  Inputs=-++
  Accelerations : Outport
  wires:
  Multiply/1 -> Sum6/2
  Gain1/1 -> Sum6/3  "acc_y"
  Sin/1 -> Multiply1/2, Gain1/1
  Derivative/1 -> Mux/1  "acc_x"
  Cos/1 -> Multiply/2, Gain2/1
  Gain2/1 -> Sum1/2  "acc_z"
  True Roll Angle/1 -> Sin/1, Cos/1
  True Velocity/1 -> Derivative/1
  Centripetal Acceleration due to Path Curvature/1 -> Multiply1/1, Multiply/1
  Multiply1/1 -> Sum1/1
  Sum1/1 -> Mux/3
  Mux/1 -> Accelerations/1
  Sum6/1 -> Mux/2
  Lateral Acceleration of the IMU due to Roll/1 -> Sum6/1, Scope2/1

== system bike_model_v1_20190531_oldmodel_positionfeedback/IMU/IMU/IMU Gyroscope ==
  True Velocity : Inport
  True Roll Angle : Inport  Port=2
  Measured Steering Angle : Inport  Port=3
  "Bike Model b " : Constant  Value=b_model
  Cos : Trigonometry  Operator=cos
  Divide : Product  Inputs=*/
  Gain : Gain  Gain=sin(lambda_model)
  Multiply : Product
  Multiply1 : Product
  Multiply2 : Product
  Mux : Mux  Inputs=3
  Sin : Trigonometry
  Tan : Trigonometry  Operator=tan
  Roll rates : Outport
  wires:
  Mux/1 -> Roll rates/1
  Tan/1 -> Multiply/1
  Gain/1 -> Tan/1
  Measured Steering Angle/1 -> Gain/1
  Cos/1 -> Multiply1/1
  True Roll Angle/1 -> Mux/1, Cos/1, Sin/1
  Sin/1 -> Multiply2/1
  True Velocity/1 -> Divide/1
  "Bike Model b "/1 -> Divide/2
  Divide/1 -> Multiply/2  "v/b"
  Multiply/1 -> Multiply2/2, Multiply1/2
  Multiply2/1 -> Mux/2
  Multiply1/1 -> Mux/3

== system bike_model_v1_20190531_oldmodel_positionfeedback/Path Tracking Controllers/Reference Position and Direction in Global CS with variable Look Ahead/Reference Position and Angle Selector ==
  total travelled distance : Inport
  1-D Lookup Table : Lookup_n-D  NumberOfTableDimensions=1  BreakpointsForDimension1=cumulative_dist_along_path  Table=path_x  ExtrapMethod=Clip  DiagnosticForOutOfRangeInput=Error  InternalRulePriority=Speed  RndMeth=Simplest  InputSameDT=on
  1-D Lookup Table1 : Lookup_n-D  NumberOfTableDimensions=1  BreakpointsForDimension1=cumulative_dist_along_path  Table=path_y  ExtrapMethod=Clip  DiagnosticForOutOfRangeInput=Error  InternalRulePriority=Speed  RndMeth=Simplest  InputSameDT=on
  Atan2 : Trigonometry  Operator=atan2
  Derivative : Derivative
  Derivative1 : Derivative
  Scope : Scope
  Unwrap : dspsigops/Unwrap  tol=pi  InputProcessing=Columns as channels (frame based)  running=off
  Zero-Order Hold : ZeroOrderHold  SampleTime=-1
  X_sigma : Outport
  Y_sigma : Outport  Port=2
  psi_sigma : Outport  Port=3
  wires:
  total travelled distance/1 -> 1-D Lookup Table1/1, 1-D Lookup Table/1
  Unwrap/1 -> Scope/1, psi_sigma/1
  1-D Lookup Table/1 -> X_sigma/1, Derivative1/1  "interpolated path x value"
  Derivative1/1 -> Atan2/2  "dx"
  Derivative/1 -> Atan2/1  "dy"
  Atan2/1 -> Zero-Order Hold/1
  1-D Lookup Table1/1 -> Y_sigma/1, Derivative/1  "interpolated path y value"
  Zero-Order Hold/1 -> Unwrap/1

== system bike_model_v1_20190531_oldmodel_positionfeedback/Path Tracking Controllers/Reference Position and Direction in Global CS with variable Look Ahead/Subsystem1 ==
  total travelled distance : Inport
  1-D Lookup Table : Lookup_n-D  NumberOfTableDimensions=1  BreakpointsForDimension1=cumulative_dist_along_path  Table=path_x  ExtrapMethod=Clip  DiagnosticForOutOfRangeInput=Error  InternalRulePriority=Speed  RndMeth=Simplest  InputSameDT=on
  1-D Lookup Table1 : Lookup_n-D  NumberOfTableDimensions=1  BreakpointsForDimension1=cumulative_dist_along_path  Table=path_y  ExtrapMethod=Clip  DiagnosticForOutOfRangeInput=Error  InternalRulePriority=Speed  RndMeth=Simplest  InputSameDT=on
  Atan2 : Trigonometry  Operator=atan2
  Derivative : Derivative
  Derivative1 : Derivative
  Scope : Scope
  Unwrap : dspsigops/Unwrap  tol=pi  InputProcessing=Columns as channels (frame based)  running=off
  Zero-Order Hold : ZeroOrderHold  SampleTime=-1
  X_sigma : Outport
  Y_sigma : Outport  Port=2
  psi_sigma : Outport  Port=3
  wires:
  total travelled distance/1 -> 1-D Lookup Table1/1, 1-D Lookup Table/1
  Unwrap/1 -> Scope/1, psi_sigma/1
  1-D Lookup Table/1 -> X_sigma/1, Derivative1/1  "interpolated path x value"
  Derivative1/1 -> Atan2/2  "dx"
  Derivative/1 -> Atan2/1  "dy"
  Atan2/1 -> Zero-Order Hold/1
  1-D Lookup Table1/1 -> Y_sigma/1, Derivative/1  "interpolated path y value"
  Zero-Order Hold/1 -> Unwrap/1

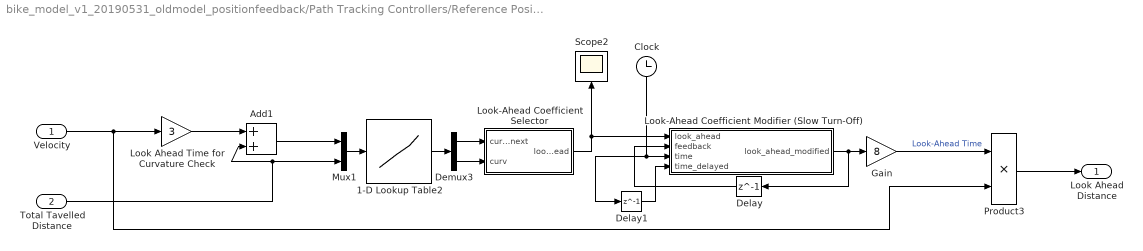
== system bike_model_v1_20190531_oldmodel_positionfeedback/Path Tracking Controllers/Reference Position and Direction in Global CS with variable Look Ahead/Variable Look Ahead ==
  Velocity : Inport
  Total Tavelled Distance : Inport  Port=2
  1-D Lookup Table2 : Lookup_n-D  NumberOfTableDimensions=1  BreakpointsForDimension1=cumulative_dist_along_path  Table=curvature  ExtrapMethod=Clip  DiagnosticForOutOfRangeInput=Error  InternalRulePriority=Speed  RndMeth=Simplest  InputSameDT=on
  Add1 : Sum
  Clock : Clock
  Delay : Delay  DelayLength=1
  Delay1 : Delay  DelayLength=1
  Demux3 : Demux  Outputs=2
  Gain : Gain  Gain=8
  Look Ahead Time for Curvature Check : Gain  Gain=3
  Look-Ahead Coefficient Selector : MATLAB Function  TreatAsAtomicUnit=on
  "Look-Ahead Coefficient Modifier (Slow Turn-Off) " : MATLAB Function  TreatAsAtomicUnit=on
  Mux1 : Mux  Inputs=2
  Product3 : Product
  Scope2 : Scope
  Look Ahead Distance : Outport
  wires:
  Look Ahead Time for Curvature Check/1 -> Add1/1
  Delay/1 -> "Look-Ahead Coefficient Modifier (Slow Turn-Off) "/2(feedback)
  "Look-Ahead Coefficient Modifier (Slow Turn-Off) "/1(look_ahead_modified) -> Delay/1, Gain/1
  Demux3/1 -> Look-Ahead Coefficient Selector/1(curv_next)
  Look-Ahead Coefficient Selector/1(look_ahead) -> "Look-Ahead Coefficient Modifier (Slow Turn-Off) "/1(look_ahead), Scope2/1
  Clock/1 -> "Look-Ahead Coefficient Modifier (Slow Turn-Off) "/3(time), Delay1/1
  Delay1/1 -> "Look-Ahead Coefficient Modifier (Slow Turn-Off) "/4(time_delayed)
  1-D Lookup Table2/1 -> Demux3/1
  Total Tavelled Distance/1 -> Add1/2, Mux1/2
  Demux3/2 -> Look-Ahead Coefficient Selector/2(curv)
  Gain/1 -> Product3/1  "Look-Ahead Time"
  Add1/1 -> Mux1/1
  Mux1/1 -> 1-D Lookup Table2/1
  Velocity/1 -> Product3/2, Look Ahead Time for Curvature Check/1
  Product3/1 -> Look Ahead Distance/1

== system bike_model_v1_20190531_oldmodel_positionfeedback/Complementary filter/Roll Angle Estimation of Accelerometer/Lateral Acceleration Compensator/Low Pass Filter ==
  Roll Rate : Inport
  Delay18 : Delay  DelayLength=1
  Gain4 : Gain  Gain=roll_rate_coef
  Gain6 : Gain  Gain=1-roll_rate_coef
  Scope7 : Scope  NumInputPorts=2
  Sum4 : Sum  Inputs=|++
  Filtered Roll Rate : Outport
  wires:
  Gain6/1 -> Sum4/1
  Gain4/1 -> Sum4/2
  Sum4/1 -> Filtered Roll Rate/1, Delay18/1, Scope7/2  "Filtered Roll Rate"
  Delay18/1 -> Gain4/1
  Roll Rate/1 -> Scope7/1, Gain6/1  "Measured Roll Rate"

== system bike_model_v1_20190531_oldmodel_positionfeedback/Complementary filter/Roll Angle Estimation of Accelerometer/Lateral Acceleration Compensator/Numerical Derivative ==
  Roll Rate : Inport
  Delay18 : Delay  DelayLength=1
  Gain3 : Gain  Gain=1/Ts_IMU
  Sum3 : Sum  Inputs=|+-
  Roll Acceleration : Outport
  wires:
  Sum3/1 -> Gain3/1
  Delay18/1 -> Sum3/2
  Roll Rate/1 -> Sum3/1, Delay18/1
  Gain3/1 -> Roll Acceleration/1

== system bike_model_v1_20190531_oldmodel_positionfeedback/Complementary filter/Roll Angle Estimation of Accelerometer/Lateral Acceleration Compensator/Subsystem ==
  In1 : Inport
  Constant : Constant  Value=A
  Constant1 : Constant  Value=B
  Delay1 : Delay  DelayLength=1  InitialCondition=[0 0 0]  SampleTime=Ts_IMU
  Multiply : Product  Multiplication=Matrix(*)
  Multiply1 : Product  Multiplication=Matrix(*)
  Sum2 : Sum  Inputs=|++
  Out1 : Outport
  wires:
  Sum2/1 -> Delay1/1
  Multiply1/1 -> Sum2/2
  In1/1 -> Multiply1/2  "u"
  Delay1/1 -> Multiply/2, Out1/1  "x"
  Multiply/1 -> Sum2/1
  Constant/1 -> Multiply/1
  Constant1/1 -> Multiply1/1

== matlab function bike_model_v1_20190531_oldmodel_positionfeedback/Balance Controller/Reference States/Reference Roll Angle Calculator ==
  data: parameters_real input; velocity input; delta_ref input; phi_ref output
function phi_ref = fcn(parameters_real, velocity, delta_ref)
g = parameters_real(1);
b = parameters_real(3);
v = velocity;

phi_ref = -atan(v^2 / (g * b) * delta_ref); % tan(theta_ref));

== matlab function bike_model_v1_20190531_oldmodel_positionfeedback/Physical Bike/Linear Bicycle Model ==
  data: states input; input input; xdot output; velocity input; disturbance input; parameters_real input
function xdot = fcn(states,input,velocity,disturbance,parameters_real)

delta_d=input;
v=velocity;
d1=disturbance(1);
d2=disturbance(2);
d3=disturbance(3);

g=parameters_real(1);
h=parameters_real(2);
b=parameters_real(3);
a=parameters_real(4);
lambda=parameters_real(5);
c=parameters_real(6);

phi=states(1);
delta=states(2);
phi_d=states(3);

xdot1=phi_d+d1;
xdot2=delta_d+d2;
xdot3=(g/h)*phi+((a*v)/(b*h))*sin(lambda)*delta_d+((h*v^2-g*a*c)/(b*h^2))*sin(lambda)*delta+d3;

xdot=[xdot1 xdot2 xdot3];

== matlab function bike_model_v1_20190531_oldmodel_positionfeedback/Path Tracking Controllers/Reference Position and Direction in Global CS with variable Look Ahead/Variable Look Ahead/Look-Ahead Coefficient Modifier (Slow Turn-Off)  ==
  data: look_ahead input; look_ahead_modified output; feedback input; time input; time_delayed input
function look_ahead_modified = fcn(look_ahead, feedback, time, time_delayed)

step=time-time_delayed;

kill_time=3;

delta=(feedback*step)/kill_time;

if look_ahead-feedback<-0.0001
    look_ahead_modified=feedback-delta;
else
    look_ahead_modified = look_ahead;
end
    

end

== matlab function bike_model_v1_20190531_oldmodel_positionfeedback/Path Tracking Controllers/Reference Position and Direction in Global CS with variable Look Ahead/Variable Look Ahead/Look-Ahead Coefficient Selector ==
  data: curv_next input; look_ahead output; curv input
function look_ahead = fcn(curv_next, curv)


if curv>-0.01 && curv<0.01
    curv=0;
end

if curv_next>-0.01 && curv_next<0.01
    curv_next=0;
end



if curv>=0
    if curv-curv_next>0
        look_ahead=0;
    else
        look_ahead=curv_next-curv;
    end
else
    if curv-curv_next<0
        look_ahead=0;
    else
        look_ahead=curv-curv_next;
    end
end



end

== matlab function bike_model_v1_20190531_oldmodel_positionfeedback/Complementary filter/Roll Angle Estimation of Accelerometer/Lateral Acceleration Compensator/Linear Bicycle Model ==
  data: states input; input input; xdot output; velocity input; parameters_model input
function xdot = fcn(states,input,velocity,parameters_model)

delta_d=input;
v=velocity;

g=parameters_model(1);
h=parameters_model(2);
b=parameters_model(3);
a=parameters_model(4);
lambda=parameters_model(5);
c=parameters_model(6);

phi=states(1);
delta=states(2);
phi_d=states(3);

xdot1=phi_d;
xdot2=delta_d;
xdot3=(g/h)*phi+((a*v)/(b*h))*sin(lambda)*delta_d+((h*v^2-g*a*c)/(b*h^2))*sin(lambda)*delta;

xdot=[xdot1 xdot2 xdot3];

== matlab function bike_model_v1_20190531_oldmodel_positionfeedback/Global Angles and Coordinates Calculator - Position/Measured Bike Angles to Global Angles/MATLAB Function ==
  data: v input; parameters_model input; delta input; psi_d output; beta output
function [psi_d, beta]  = fcn(v, parameters_model, delta)

b = parameters_model(3);
a = parameters_model(4);

beta = atan((a / (b)) * tan(delta));
psi_d = (v / a) * sin(beta);

== matlab function bike_model_v1_20190531_oldmodel_positionfeedback/Physical Bike/Nonlinear Bicycle Model ==
  data: states input; input input; xdot output; velocity input; disturbance input; parameters_real input
function xdot = fcn(states,input,velocity,disturbance,parameters_real)

delta_d=input;
v=velocity;
d1=disturbance(1);
d2=disturbance(2);
d3=disturbance(3);

g=parameters_real(1);
h=parameters_real(2);
b=parameters_real(3);
a=parameters_real(4);
lambda=parameters_real(5);
c=parameters_real(6);

phi=states(1);
delta=states(2);
phi_d=states(3);

xdot1=phi_d+d1;
xdot2=delta_d+d2;
xdot3=(g/h)*tan(phi)+((a*v)/(b*h))*sin(lambda)*tan(delta_d)+((h*v^2-g*a*c)/(b*h^2))*sin(lambda)*tan(delta)+d3;

xdot=[xdot1 xdot2 xdot3];

== matlab function bike_model_v1_20190531_oldmodel_positionfeedback/Physical Bike/Linear Bicycle Model with neglected fork angle (lambda=90deg, c=0) "THE SIMPLEST MODEL" ==
  data: states input; input input; xdot output; velocity input; disturbance input; parameters_real input
function xdot = fcn(states,input,velocity,disturbance,parameters_real)

delta_d=input;
v=velocity;
d1=disturbance(1);
d2=disturbance(2);
d3=disturbance(3);

g=parameters_real(1);
h=parameters_real(2);
b=parameters_real(3);
a=parameters_real(4);

phi=states(1);
delta=states(2);
phi_d=states(3);

xdot1=phi_d+d1;
xdot2=delta_d+d2;
xdot3=(g/h)*phi+((a*v)/(b*h))*delta_d+((v^2)/(b*h))*delta+d3;

xdot=[xdot1 xdot2 xdot3];

== matlab function bike_model_v1_20190531_oldmodel_positionfeedback/Global Angles and Coordinates Calculator - Velocity/Measured Bike Angles to Global Angles/MATLAB Function ==
  data: v input; parameters_model input; delta input; psi_d output; beta output
function [psi_d, beta]  = fcn(v, parameters_model, delta)

b = parameters_model(3);
a = parameters_model(4);

beta = atan((a / (b)) * tan(delta));
psi_d = (v / a) * sin(beta);

== matlab function bike_model_v1_20190531_oldmodel_positionfeedback/Complementary filter/Roll Angle Estimation of Accelerometer/Lateral Acceleration Compensator/Linear Bicycle Model1 ==
  data: states input; input input; xdot output; velocity input; parameters_model input
function xdot = fcn(states,input,velocity,parameters_model)

delta_d=input;
v=velocity;

g=parameters_model(1);
h=parameters_model(2);
b=parameters_model(3);
a=parameters_model(4);
lambda=parameters_model(5);
c=parameters_model(6);

phi=states(1);
delta=states(2);
phi_d=states(3);

xdot1=phi_d;
xdot2=delta_d;
xdot3=(g/h)*phi+((a*v)/(b*h))*sin(lambda)*delta_d+((h*v^2-g*a*c)/(b*h^2))*sin(lambda)*delta;

xdot=[xdot1; xdot2; xdot3];

== matlab function bike_model_v1_20190531_oldmodel_positionfeedback/Complementary filter/Roll Angle Estimation of Accelerometer/Lateral Acceleration Compensator/discrete ==
  data: states input; input input; x_next output; A input; B input
function x_next = fcn(states,input,A,B)





x_next=A*states+B*input;

== matlab function bike_model_v1_20190531_oldmodel_positionfeedback/Global Angles and Coordinates Calculator - Velocity/Measured Global Angles to Global Coordinates/MATLAB Function1 ==
  data: v input; psi input; Xdot output; beta input; Ydot output
function [Xdot, Ydot]  = fcn(v, psi, beta)

Xdot = v * cos(psi + beta);
Ydot = v * sin(psi + beta);

== matlab function bike_model_v1_20190531_oldmodel_positionfeedback/Global Angles and Coordinates Calculator - Position/Measured Global Angles to Global Coordinates/MATLAB Function1 ==
  data: v input; psi input; Xdot output; beta input; Ydot output
function [Xdot, Ydot]  = fcn(v, psi, beta)

Xdot = v * cos(psi + beta);
Ydot = v * sin(psi + beta);
